simulink model "optotrack_odometry_comp"  (R2019b)
settings: Solver=FixedStepDiscrete  StartTime=0.0  StopTime=inf  FixedStep=1/100  RelTol=1e-3
libraries: dspnetwork x2
settings Model: EnablePacing=on  Creator=student  LastModifiedBy=student

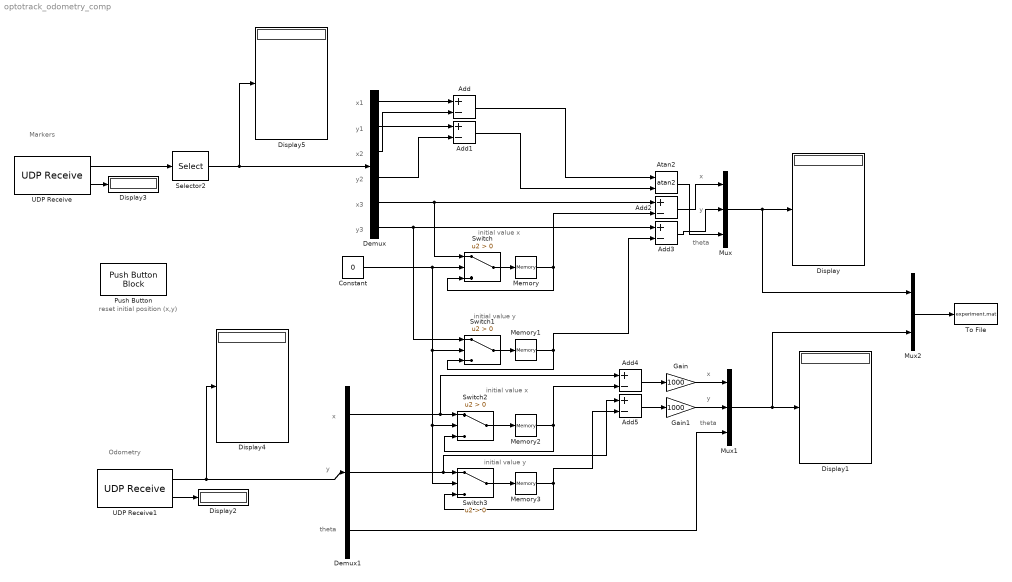
== system optotrack_odometry_comp ==
  note: reset initial position (x,y)
  note: theta
  note: y
  note: x
  note: y
  note: initial value x
  note: theta
  note: y3
  note: x3
  note: y2
  note: x2
  note: y1
  note: x1
  note: Markers
  note: Odometry
  note: initial value y
  note: x
  note: initial value x
  note: initial value y
  note: x
  note: y
  note: theta
  Add{,1..5} (6 alike) : Sum  Inputs=+-
  Atan2 : Trigonometry  Operator=atan2
  Constant : Constant  Value=0
  Demux : Demux  Outputs=6
  Demux1 : Demux  Outputs=3
  Display{,1..5} (6 alike) : Display
  Gain : Gain  Gain=1000
  Gain1 : Gain  Gain=1000
  Memory{,1..3} (4 alike) : Memory
  Mux : Mux  Inputs=3
  Mux1 : Mux  Inputs=3
  Mux2 : Mux  Inputs=2
  Push Button : PushButtonBlock
  Selector2 : Selector  InputPortWidth=9  IndexOptions=Index vector (dialog)  Indices=[1 2 4 5 7 8]  OutputSizes=1
  Switch{,1..3} (4 alike) : Switch  Criteria=u2 > Threshold
  To File : ToFile  Filename=experiment.mat  SaveFormat=Timeseries
  UDP Receive : dspnetwork/UDP Receive  localURL='0.0.0.0'  localPort=25000  remoteURL='0.0.0.0'  remotePort=-1  recvBufferSize=3*3*4  dims=3*3  signalDatatype=single  isComplex=off  isVarSize=off  showBlockingTime=off  blockingTime=0  sampletime=1/100  blockPlatform=[]
      settings: SourceProductName=Simulink
  UDP Receive1 : dspnetwork/UDP Receive  localURL='0.0.0.0'  localPort=5001  remoteURL='0.0.0.0'  remotePort=-1  recvBufferSize=3*4  dims=3  signalDatatype=single  isComplex=off  isVarSize=off  showBlockingTime=off  blockingTime=0  sampletime=1/100  blockPlatform=[]
      settings: SourceProductName=Simulink
  wires:
  UDP Receive/1 -> Selector2/1
  Demux/1 -> Add/1
  Demux/3 -> Add/2
  Demux/2 -> Add1/1
  Demux/4 -> Add1/2
  Switch/1 -> Memory/1
  Switch1/1 -> Memory1/1
  Memory/1 -> Add2/2, Switch/3
  Memory1/1 -> Switch1/3, Add3/2
  Demux/5 -> Switch/1, Add2/1
  Demux/6 -> Switch1/1, Add3/1
  Constant/1 -> Switch3/2, Switch2/2, Switch1/2, Switch/2
  UDP Receive1/1 -> Display4/1, Demux1/1
  Switch2/1 -> Memory2/1
  Memory2/1 -> Switch2/3, Add4/2
  Memory3/1 -> Switch3/3, Add5/2
  Switch3/1 -> Memory3/1
  Demux1/2 -> Add5/1, Switch3/1
  Demux1/1 -> Add4/1, Switch2/1
  Atan2/1 -> Mux/3
  Add2/1 -> Mux/1
  Add3/1 -> Mux/2
  Demux1/3 -> Mux1/3
  Mux1/1 -> Mux2/2, Display1/1
  Mux/1 -> Mux2/1, Display/1
  UDP Receive1/2 -> Display2/1
  UDP Receive/2 -> Display3/1
  Selector2/1 -> Display5/1, Demux/1
  Add/1 -> Atan2/1
  Add1/1 -> Atan2/2
  Mux2/1 -> To File/1
  Add4/1 -> Gain/1
  Gain/1 -> Mux1/1
  Gain1/1 -> Mux1/2
  Add5/1 -> Gain1/1
